simulink model "LAB7_PI"  (R2022b)
settings: Solver=VariableStepAuto  StartTime=0.0  StopTime=czas_systemu  RelTol=1e-3
values from neighbouring files (symbols this model uses):
  Cvp = cp*rop*Vp    (= 48000)    [LAB7.m]
  Cvw = cp*rop*Vw    (= 67200)    [LAB7.m]
  dqg = 0.1*q_g_N    (= 1000)    [LAB7.m]
  dTzew = 1    [LAB7.m]
  K_cp = ((a1*q_g_N)*(T_wew_N-Tp_N))/((Tp_N-T_zew_N)*(T_wew_N-T_zew_N+a1*(T_wew_N-Tp_N)))    (= 23.2558139535)    [LAB7.m]
  K_cw = (q_g_N)/(T_wew_N-T_zew_N+a1*(T_wew_N-Tp_N))    (= 232.558139535)    [LAB7.m]
  K_cwp = (a1*(q_g_N))/(T_wew_N-T_zew_N+a1*(T_wew_N-Tp_N))    (= 69.7674418605)    [LAB7.m]
  Kd = 0    [LAB7.m]
  Ki = 1/0.1129    (= 8.8573959256)    [LAB7.m]
  Kp = 2948    [LAB7.m]
  L11 = [ksTwew]    [LAB7.m]
  L12 = [ksTp]    [LAB7.m]
  L21 = [kmdTwew]    [LAB7.m]
  L22 = [kmdTp]    [LAB7.m]
  M1 = [T,1]    [LAB7.m]
  M2 = [T_sp,1]    [LAB7.m]
  M3 = [T2,1]    [LAB7.m]
  M4 = [T3,1]    [LAB7.m]
  q_g_0 = K_cw*(T_wew_0-T_zew_0)-K_cwp*(T_wew_0-Tp_0)    (= 9178.29457364)    [LAB7.m]
  t0 = 0    [LAB7.m]
  T_0_tp = 100    [LAB7.m]
  T_0_wew = 0    [LAB7.m]
  T_wew_0 = (K_cwp*Tp_0+K_cp*(Tp_0-T_zew_0))/K_cwp    (= 22.6666666667)    [LAB7.m]
  T_zew_0 = T_zew_N    (= -20)    [LAB7.m]
  To = t_2w-T2    (= 0)    [LAB7.m]
  To1 = t_2p-T3    (= 175)    [LAB7.m]
  Tp_0 = 12    [LAB7.m]
  Tp_N = 10    [LAB7.m]
settings Model: Creator=maciejrudy  LastModifiedBy=Dawid
settings SolverCC: AlgebraicLoopSolver=TrustRegion
settings DataIOCC: ReturnWorkspaceOutputs=off
settings DebuggingCC: UnconnectedInputMsg=warning  UnconnectedOutputMsg=warning  UnconnectedLineMsg=warning  SFMachineParentedDataDiag=warning
settings ModelReferenceCC: EnableRefExpFcnMdlSchedulingChecks=on
settings RTWCC: DLArmComputeVersion=19.05

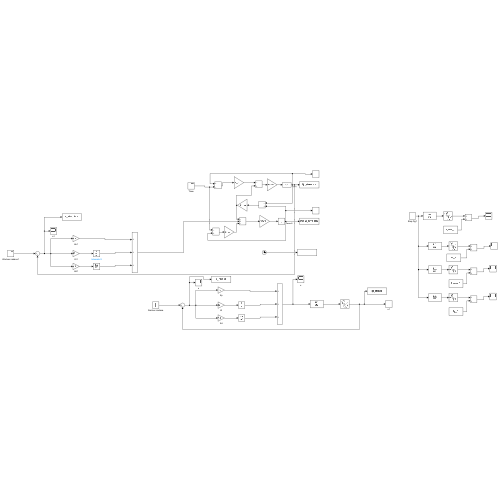
[thumbnail: Simulink's stored preview of the top-level diagram]
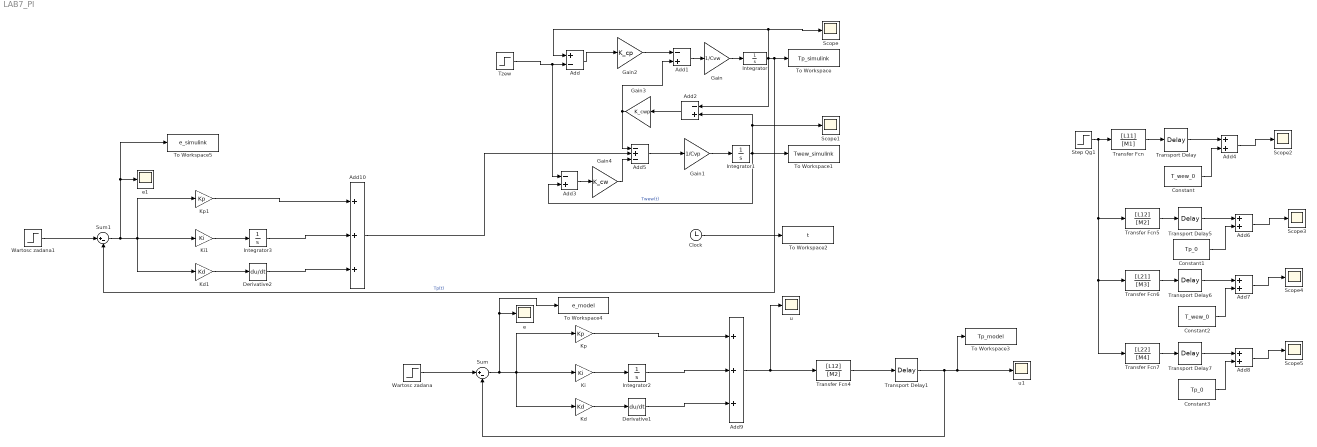
== system LAB7_PI ==
  Add : Sum  Inputs=+-
  Add1 : Sum  Inputs=-+
  Add10 : Sum  Inputs=+++
  Add2 : Sum  Inputs=-+
  Add3 : Sum  Inputs=-+
  Add{4,6..8} (4 alike) : Sum
  Add5 : Sum  Inputs=-+-
  Add9 : Sum  Inputs=+++
  Clock : Clock
  Constant : Constant  Value=T_wew_0
  Constant1 : Constant  Value=Tp_0
  Constant2 : Constant  Value=T_wew_0
  Constant3 : Constant  Value=Tp_0
  Derivative1 : Derivative
  Derivative2 : Derivative
  Gain : Gain  Gain=1/Cvw
  Gain1 : Gain  Gain=1/Cvp
  Gain2 : Gain  Gain=K_cp
  Gain3 : Gain  Gain=K_cwp
  Gain4 : Gain  Gain=K_cw
  Integrator : Integrator  InitialCondition=Tp_0
  Integrator1 : Integrator  InitialCondition=T_wew_0
  Integrator2 : Integrator  InitialCondition=q_g_0
  Integrator3 : Integrator  InitialCondition=q_g_0
  Kd : Gain  Gain=Kd
  Kd1 : Gain  Gain=Kd
  Ki : Gain  Gain=Ki
  Ki1 : Gain  Gain=Ki
  Kp : Gain  Gain=Kp
  Kp1 : Gain  Gain=Kp
  Scope{,1..5} (6 alike) : Scope
  Step Qg1 : Step  Time=t0  After=dqg  SampleTime=0
  Sum : Sum  Inputs=|+-
  Sum1 : Sum  Inputs=|+-
  To Workspace : ToWorkspace  VariableName=Tp_simulink  SampleTime=-1
  To Workspace1 : ToWorkspace  VariableName=Twew_simulink  SampleTime=-1
  To Workspace2 : ToWorkspace  VariableName=t  SaveFormat=Timeseries  SampleTime=-1
  To Workspace3 : ToWorkspace  VariableName=Tp_model  SampleTime=-1
  To Workspace4 : ToWorkspace  VariableName=e_model  SampleTime=-1
  To Workspace5 : ToWorkspace  VariableName=e_simulink  SampleTime=-1
  Transfer Fcn : TransferFcn  Numerator=[L11]  Denominator=[M1]
  Transfer Fcn4 : TransferFcn  Numerator=[L12]  Denominator=[M2]
  Transfer Fcn5 : TransferFcn  Numerator=[L12]  Denominator=[M2]
  Transfer Fcn6 : TransferFcn  Numerator=[L21]  Denominator=[M3]
  Transfer Fcn7 : TransferFcn  Numerator=[L22]  Denominator=[M4]
  Transport Delay : TransportDelay  DelayTime=T_0_wew
  Transport Delay1 : TransportDelay  DelayTime=T_0_tp
  Transport Delay5 : TransportDelay  DelayTime=T_0_tp
  Transport Delay6 : TransportDelay  DelayTime=To
  Transport Delay7 : TransportDelay  DelayTime=To1
  Tzew : Step  Time=t0  Before=T_zew_0  After=T_zew_0+dTzew  SampleTime=0
  Wartosc zadana : Step  Time=t0  Before=Tp_N  After=Tp_0  SampleTime=0
  Wartosc zadana1 : Step  Time=t0  After=12  SampleTime=0
  e : Scope
  e1 : Scope
  u : Scope
  u1 : Scope
  wires:
  Wartosc zadana/1 -> Sum/1
  Transfer Fcn4/1 -> Transport Delay1/1
  Transport Delay6/1 -> Add7/1
  Add9/1 -> u/1, Transfer Fcn4/1
  Gain3/1 -> Add5/1, Add1/2
  Add4/1 -> Scope2/1
  Gain/1 -> Integrator/1
  Transport Delay7/1 -> Add8/1
  Add2/1 -> Gain3/1
  Constant1/1 -> Add6/2
  Add5/1 -> Gain1/1
  Constant/1 -> Add4/2
  Gain4/1 -> Add5/3
  Gain1/1 -> Integrator1/1
  Integrator/1 -> Add2/1, To Workspace/1, Sum1/2, Scope/1, Add/1  "Tp(t)"
  Transfer Fcn5/1 -> Transport Delay5/1
  Add8/1 -> Scope5/1
  Add1/1 -> Gain/1
  Transport Delay/1 -> Add4/1
  Step Qg1/1 -> Transfer Fcn5/1, Transfer Fcn7/1, Transfer Fcn6/1, Transfer Fcn/1
  Transfer Fcn7/1 -> Transport Delay7/1
  Clock/1 -> To Workspace2/1
  Add/1 -> Gain2/1
  Integrator1/1 -> Add3/2, To Workspace1/1, Add2/2, Scope1/1  "Twew(t)"
  Add3/1 -> Gain4/1
  Transport Delay5/1 -> Add6/1
  Constant2/1 -> Add7/2
  Transfer Fcn/1 -> Transport Delay/1
  Add7/1 -> Scope4/1
  Tzew/1 -> Add3/1, Add/2
  Constant3/1 -> Add8/2
  Ki/1 -> Integrator2/1
  Add6/1 -> Scope3/1
  Gain2/1 -> Add1/1
  Integrator2/1 -> Add9/2
  Transfer Fcn6/1 -> Transport Delay6/1
  Sum/1 -> To Workspace4/1, e/1, Ki/1, Kp/1, Kd/1
  Kp/1 -> Add9/1
  Kd/1 -> Derivative1/1
  Derivative1/1 -> Add9/3
  Transport Delay1/1 -> Sum/2, u1/1, To Workspace3/1
  Sum1/1 -> To Workspace5/1, e1/1, Ki1/1, Kp1/1, Kd1/1
  Integrator3/1 -> Add10/2
  Kd1/1 -> Derivative2/1
  Derivative2/1 -> Add10/3
  Kp1/1 -> Add10/1
  Ki1/1 -> Integrator3/1
  Wartosc zadana1/1 -> Sum1/1
  Add10/1 -> Add5/2
